simulink model "speakerModel"  (R2018b)
settings: Solver=VariableStepAuto  StartTime=0.0  StopTime=10.0  RelTol=1e-3
settings Model: Creator=jpedley  LastModifiedBy=james

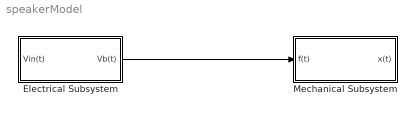
== system speakerModel ==
  Electrical Subsystem : Subsystem
  Mechanical Subsystem : Subsystem
  wires:
  Electrical Subsystem/1(Vb(t)) -> Mechanical Subsystem/1(f(t))

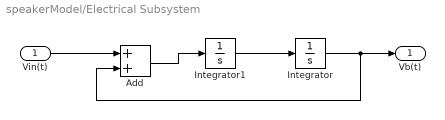
== system speakerModel/Electrical Subsystem ==
  Vin(t) : Inport
  Add : Sum
  Integrator : Integrator
  Integrator1 : Integrator
  Vb(t) : Outport  VectorParamsAs1DForOutWhenUnconnected=off
  wires:
  Vin(t)/1 -> Add/1
  Add/1 -> Integrator1/1
  Integrator/1 -> Add/2, Vb(t)/1
  Integrator1/1 -> Integrator/1

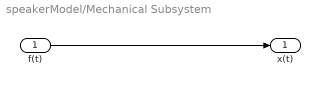
== system speakerModel/Mechanical Subsystem ==
  f(t) : Inport
  x(t) : Outport  VectorParamsAs1DForOutWhenUnconnected=off
  wires:
  f(t)/1 -> x(t)/1
